simulink model "mbed_nucleo_f303_spi_peripherals"  (R2015a)
settings: Solver=FixedStepDiscrete  SolverMode=SingleTasking  StartTime=0.0  StopTime=10.0  FixedStep=1  RelTol=1e-3
undefined symbols (not defined in the file or in its folder): Ended, Single, x2
libraries: mbed_lib x15, simulink x3, mbed_targets_stm_disco_f407 x2, mbed_targets_stm_nucleo_f303 x1
settings Model: Creator=Stuv  LastModifiedBy=Stuv
settings OptimizationCC: OptimizeModelRefInitCode=on  LifeSpan=1
settings HardwareCC: ProdLargestAtomicInteger=Long  ProdLargestAtomicFloat=Double  ProdEndianess=LittleEndian  ProdHWDeviceType=ARM Compatible->ARM Cortex
settings RTWCC: SystemTargetFile=mbed.tlc  TemplateMakefile=mbed.tmf  Description=Mbed Target (Embedded Target)  TargetLang=C++
settings CodeAppCC: IgnoreCustomStorageClasses=off
settings STFCustomTargetCC: CombineOutputUpdateFcns=on  SupportContinuousTime=off  SupportVariableSizeSignals=off  SystemTargetFile=mbed.tlc
settings ERTTargetCC: SupportContinuousTime=off  SupportVariableSizeSignals=off  ERTCustomFileTemplate=mbed_file_process.tlc

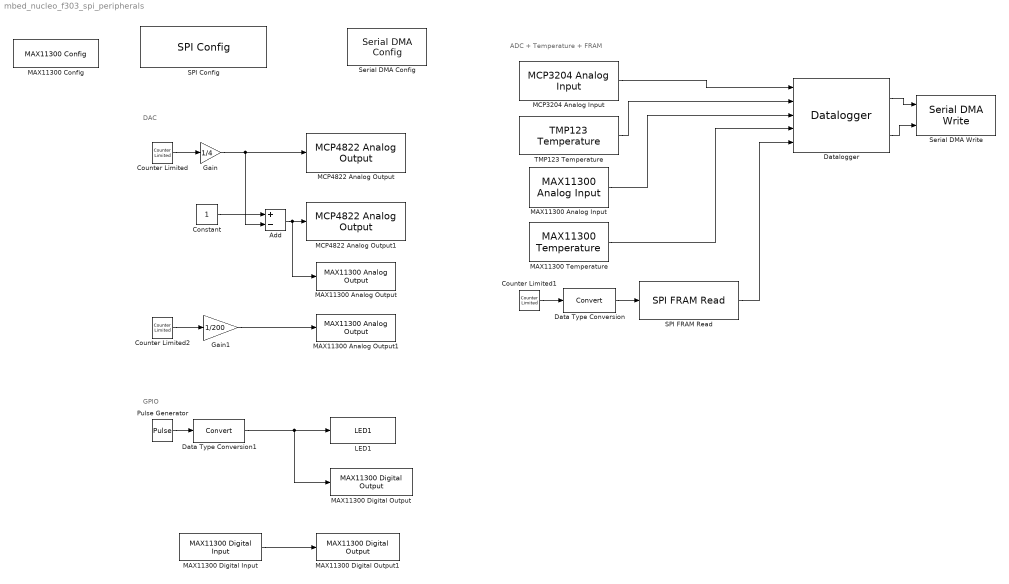
== system mbed_nucleo_f303_spi_peripherals ==
  note: GPIO
  note: DAC
  note: ADC + Temperature + FRAM
  Add : Sum  Inputs=+-
  Constant : Constant  OutDataTypeStr=single
  Counter Limited : simulink/Sources/Counter Limited  uplimit=4  tsamp=-1
  Counter Limited1 : simulink/Sources/Counter Limited  uplimit=12  tsamp=-1
  Counter Limited2 : simulink/Sources/Counter Limited  uplimit=100  tsamp=-1
  Data Type Conversion : DataTypeConversion
  Data Type Conversion1 : DataTypeConversion
  Datalogger : mbed_lib/Utilities/Datalogger  TypeInputPorts={ 'single' 1 'single' 1 'single' 1 'single' 1 'uint8' 1 }  TypeOfInputs={'1*single','1*single','1*single','1*single','1*uint8'}  BufferSize=70  errEn=off  SampleTime=-1
  Gain : Gain  Gain=1/4  OutDataTypeStr=single
  Gain1 : Gain  Gain=1/200  OutDataTypeStr=single
  LED1 : mbed_targets_stm_nucleo_f303/LED1  Parameter1=0
  MAX11300 Analog Input : mbed_lib/SPI/MAX11300 Analog Input  CsPort=B  CsPin=1  InputType=Single-Ended  Mode=relative  PosPin=0  NegPin=0  Power=1  Range=-5 to +5  Ref=Internal (2.5 V)
  MAX11300 Analog Output : mbed_lib/SPI/MAX11300 Analog Output  CsPort=B  CsPin=1  Pin=1  Mode=relative  Range=0 to +10 V
  MAX11300 Analog Output1 : mbed_lib/SPI/MAX11300 Analog Output  CsPort=B  CsPin=1  Pin=5  Mode=relative  Range=0 to +10 V
  MAX11300 Config : mbed_lib/SPI/MAX11300 Config  Priority=1  SpiPort=1  CsPort=B  CsPin=1  AdcRate=400 kSPS  DacRef=Internal (2.5 V)  TempCh0=on  TempCh1=off  TempCh2=off
  MAX11300 Digital Input : mbed_lib/SPI/MAX11300 Digital Input  CsPort=B  CsPin=1  Pin=2  Thresh=4095
  MAX11300 Digital Output : mbed_lib/SPI/MAX11300 Digital Output  CsPort=B  CsPin=1  Pin=3  Level=2^12-1
  MAX11300 Digital Output1 : mbed_lib/SPI/MAX11300 Digital Output  CsPort=B  CsPin=1  Pin=4  Level=2^12-1
  MAX11300 Temperature : mbed_lib/SPI/MAX11300 Temperature  CsPort=B  CsPin=1  Channel=Internal
  MCP3204 Analog Input : mbed_lib/SPI/MCP3204 Analog Input  SpiPort=1  CsPort=A  CsPin=12  Channel=1  Mode=relative  InputType=Single ended
  MCP4822 Analog Output : mbed_lib/SPI/MCP4822 Analog Output  SpiPort=1  CsPort=A  CsPin=11  Channel=A  Mode=relative  Gain=x2
  MCP4822 Analog Output1 : mbed_lib/SPI/MCP4822 Analog Output  SpiPort=1  CsPort=A  CsPin=11  Channel=B  Mode=relative  Gain=x2
  Pulse Generator : DiscretePulseGenerator  PulseType=Time based  PulseWidth=50
  SPI Config : mbed_lib/SPI/SPI Config  Priority=0  SpiPort=1  SParameter6=1000000  SParameter2=B  SParameter3=15  SParameter4=B  SParameter5=14  SCK_PORT=B  SCK_PIN=13
  SPI FRAM Read : mbed_lib/SPI/SPI FRAM Read  SpiPort=1  CsPort=B  CsPin=12
  Serial DMA Config : mbed_targets_stm_disco_f407/Serial DMA Config  SerialPort=2  TxPort=A  TxPin=2  RxPort=A  RxPin=3  BaudRate=115200
  Serial DMA Write : mbed_targets_stm_disco_f407/Serial DMA Write  SerialPort=2  numData=on  SampleTime=-1
  TMP123 Temperature : mbed_lib/SPI/TMP123 Temperature  SpiPort=1  CsPort=B  CsPin=11
  wires:
  Datalogger/1 -> Serial DMA Write/1
  Datalogger/2 -> Serial DMA Write/2
  MCP3204 Analog Input/1 -> Datalogger/1
  TMP123 Temperature/1 -> Datalogger/2
  Counter Limited/1 -> Gain/1
  Gain/1 -> MCP4822 Analog Output/1, Add/2
  Constant/1 -> Add/1
  Add/1 -> MAX11300 Analog Output/1, MCP4822 Analog Output1/1
  SPI FRAM Read/1 -> Datalogger/5
  Counter Limited1/1 -> Data Type Conversion/1
  Data Type Conversion/1 -> SPI FRAM Read/1
  Pulse Generator/1 -> Data Type Conversion1/1
  Data Type Conversion1/1 -> MAX11300 Digital Output/1, LED1/1
  MAX11300 Analog Input/1 -> Datalogger/3
  MAX11300 Temperature/1 -> Datalogger/4
  MAX11300 Digital Input/1 -> MAX11300 Digital Output1/1
  Counter Limited2/1 -> Gain1/1
  Gain1/1 -> MAX11300 Analog Output1/1
